simulink library "util_tf_lib"  (R2014b)
settings: Solver=ode45  SolverMode=SingleTasking  StartTime=0.0  StopTime=10.0  RelTol=1e-3
settings Model: Creator=hcannon  LastModifiedBy=mstewart

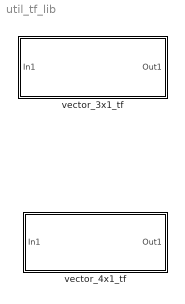
== system util_tf_lib ==
  vector_3x1_tf : Subsystem  mask{num=[1 1], den=[1 1], st=-1}
      mask prompts: num "numerator"; den "denominator"; st "sample_time"
      mask Display:
      | disp('tf')
      | color('blue')
      | text(0.05,0.02,'NASA',...
      |  	'HorizontalAlignment','Left',...
      | 	'VerticalAlignment','bottom')
  vector_4x1_tf : Subsystem  mask{num=[1 1], den=[1 1], st=-1}
      mask prompts: num "numerator"; den "denominator"; st "sample time"
      mask Display:
      | disp('tf')
      | color('blue')
      | text(0.05,0.02,'NASA',...
      |  	'HorizontalAlignment','Left',...
      | 	'VerticalAlignment','bottom')

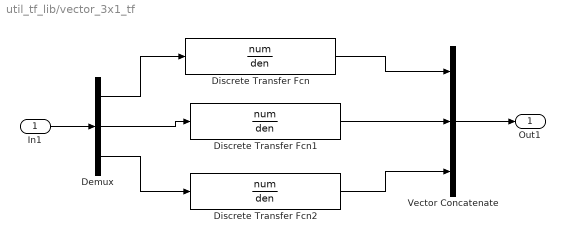
== system util_tf_lib/vector_3x1_tf ==
  In1 : Inport
  Demux : Demux  Outputs=3
  Discrete Transfer Fcn : DiscreteTransferFcn  Numerator=num  Denominator=den  SampleTime=st
  Discrete Transfer Fcn1 : DiscreteTransferFcn  Numerator=num  Denominator=den  SampleTime=st
  Discrete Transfer Fcn2 : DiscreteTransferFcn  Numerator=num  Denominator=den  SampleTime=st
  Vector Concatenate : Concatenate  NumInputs=3
  Out1 : Outport
  wires:
  In1/1 -> Demux/1
  Demux/1 -> Discrete Transfer Fcn/1
  Demux/2 -> Discrete Transfer Fcn1/1
  Demux/3 -> Discrete Transfer Fcn2/1
  Discrete Transfer Fcn/1 -> Vector Concatenate/1
  Discrete Transfer Fcn1/1 -> Vector Concatenate/2
  Discrete Transfer Fcn2/1 -> Vector Concatenate/3
  Vector Concatenate/1 -> Out1/1

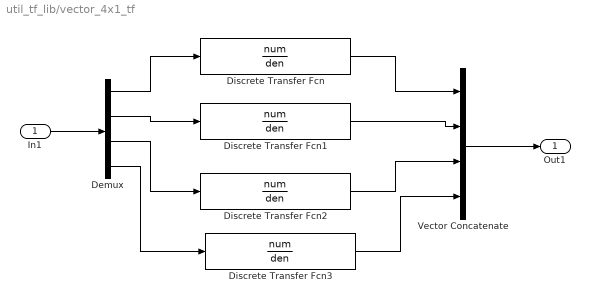
== system util_tf_lib/vector_4x1_tf ==
  In1 : Inport
  Demux : Demux
  Discrete Transfer Fcn{,1..3} (4 alike) : DiscreteTransferFcn  Numerator=num  Denominator=den  SampleTime=st
  Vector Concatenate : Concatenate  NumInputs=4
  Out1 : Outport
  wires:
  Vector Concatenate/1 -> Out1/1
  Discrete Transfer Fcn2/1 -> Vector Concatenate/3
  Discrete Transfer Fcn1/1 -> Vector Concatenate/2
  Discrete Transfer Fcn/1 -> Vector Concatenate/1
  Demux/3 -> Discrete Transfer Fcn2/1
  Demux/2 -> Discrete Transfer Fcn1/1
  Demux/1 -> Discrete Transfer Fcn/1
  In1/1 -> Demux/1
  Demux/4 -> Discrete Transfer Fcn3/1
  Discrete Transfer Fcn3/1 -> Vector Concatenate/4
